simulink model "CC3"  (Simulink 7.5)
settings: Solver=ode45  StartTime=0.0  StopTime=2  RelTol=1e-3
(part 2 of 2)

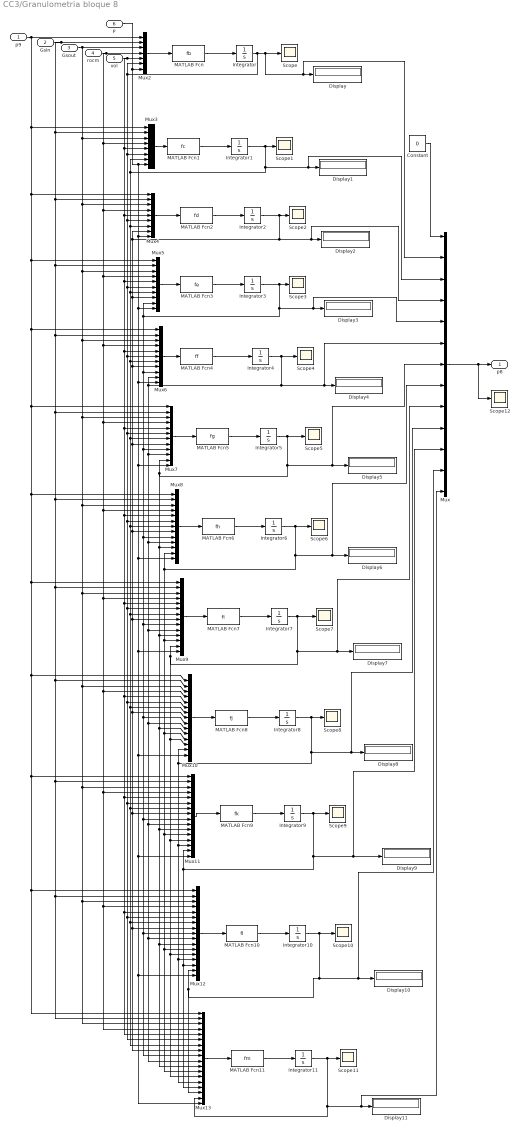
== system CC3/Granulometria bloque 8 ==
  p9 : Inport
  Gsin : Inport  Port=2
  Gsout : Inport  Port=3
  rocm : Inport  Port=4
  vol : Inport  Port=5
  P : Inport  Port=6
  Constant : Constant  Value=0  OutDataType=fixdt(1, 16)  OutScaling=2^0
  Display{,1..11} (12 alike) : Display
  Integrator{,1..11} (12 alike) : Integrator  InitialCondition=0.003
  MATLAB Fcn : MATLABFcn  MATLABFcn=fb
  MATLAB Fcn1 : MATLABFcn  MATLABFcn=fc
  MATLAB Fcn10 : MATLABFcn  MATLABFcn=fl
  MATLAB Fcn11 : MATLABFcn  MATLABFcn=fm
  MATLAB Fcn2 : MATLABFcn  MATLABFcn=fd
  MATLAB Fcn3 : MATLABFcn  MATLABFcn=fe
  MATLAB Fcn4 : MATLABFcn  MATLABFcn=ff
  MATLAB Fcn5 : MATLABFcn  MATLABFcn=fg
  MATLAB Fcn6 : MATLABFcn  MATLABFcn=fh
  MATLAB Fcn7 : MATLABFcn  MATLABFcn=fi
  MATLAB Fcn8 : MATLABFcn  MATLABFcn=fj
  MATLAB Fcn9 : MATLABFcn  MATLABFcn=fk
  Mux : Mux  Inputs=13
  Mux10 : Mux  Inputs=15
  Mux11 : Mux  Inputs=16
  Mux12 : Mux  Inputs=17
  Mux13 : Mux  Inputs=18
  Mux2 : Mux  Inputs=7
  Mux3 : Mux  Inputs=8
  Mux4 : Mux  Inputs=9
  Mux5 : Mux  Inputs=10
  Mux6 : Mux  Inputs=11
  Mux7 : Mux  Inputs=12
  Mux8 : Mux  Inputs=13
  Mux9 : Mux  Inputs=14
  Scope{,1..12} (13 alike) : Scope
      Scope settings: SaveName=ScopeData2
      Scope1 settings: SaveName=ScopeData20
      Scope10 settings: SaveName=ScopeData29
      Scope11 settings: SaveName=ScopeData30
      Scope12 settings: SaveName=ScopeData32
      Scope2 settings: SaveName=ScopeData21
      Scope3 settings: SaveName=ScopeData22
      Scope4 settings: SaveName=ScopeData23
      Scope5 settings: SaveName=ScopeData24
      Scope6 settings: SaveName=ScopeData25
      Scope7 settings: SaveName=ScopeData26
      Scope8 settings: SaveName=ScopeData27
      Scope9 settings: SaveName=ScopeData28
  p8 : Outport  OutDataType=fixdt(1, 16)  OutScaling=2^0
  wires:
  Mux2/1 -> MATLAB Fcn/1
  MATLAB Fcn/1 -> Integrator/1
  Integrator/1 -> Mux2/6, Mux3/6, Mux4/6, Mux5/6, Mux6/6, Mux7/6, Mux8/6, Mux9/6, Mux10/6, Mux11/6, Mux12/6, Mux13/6, Scope/1, Display/1, Mux/2
  p9/1 -> Mux2/1, Mux3/1, Mux4/1, Mux5/1, Mux6/1, Mux7/1, Mux8/1, Mux9/1, Mux10/1, Mux11/1, Mux12/1, Mux13/1
  Gsin/1 -> Mux2/2, Mux3/2, Mux4/2, Mux5/2, Mux6/2, Mux7/2, Mux8/2, Mux9/2, Mux10/2, Mux11/2, Mux12/2, Mux13/2
  Gsout/1 -> Mux2/3, Mux3/3, Mux4/3, Mux5/3, Mux6/3, Mux7/3, Mux8/3, Mux9/3, Mux10/3, Mux11/3, Mux12/3, Mux13/3
  rocm/1 -> Mux2/4, Mux3/4, Mux4/4, Mux5/4, Mux6/4, Mux7/4, Mux8/4, Mux9/4, Mux10/4, Mux11/4, Mux12/4, Mux13/4
  vol/1 -> Mux2/5, Mux3/5, Mux4/5, Mux5/5, Mux6/5, Mux7/5, Mux8/5, Mux9/5, Mux10/5, Mux11/5, Mux12/5, Mux13/5
  Mux3/1 -> MATLAB Fcn1/1
  MATLAB Fcn1/1 -> Integrator1/1
  Integrator1/1 -> Scope1/1, Mux3/7, Mux4/7, Mux5/7, Mux6/7, Mux7/7, Mux8/7, Mux9/7, Mux10/7, Mux11/7, Mux12/7, Mux13/7, Display1/1, Mux/3
  Mux4/1 -> MATLAB Fcn2/1
  MATLAB Fcn2/1 -> Integrator2/1
  Integrator2/1 -> Scope2/1, Mux4/8, Mux5/8, Mux6/8, Mux7/8, Mux8/8, Mux9/8, Mux10/8, Mux11/8, Mux12/8, Mux13/8, Display2/1, Mux/4
  MATLAB Fcn3/1 -> Integrator3/1
  Integrator3/1 -> Scope3/1, Mux5/9, Mux6/9, Mux7/9, Mux8/9, Mux9/9, Mux10/9, Mux11/9, Mux12/9, Mux13/9, Display3/1, Mux/5
  Mux5/1 -> MATLAB Fcn3/1
  Mux6/1 -> MATLAB Fcn4/1
  MATLAB Fcn4/1 -> Integrator4/1
  Integrator4/1 -> Scope4/1, Mux6/10, Mux7/10, Mux8/10, Mux9/10, Mux10/10, Mux11/10, Mux12/10, Mux13/10, Display4/1, Mux/6
  Mux7/1 -> MATLAB Fcn5/1
  MATLAB Fcn5/1 -> Integrator5/1
  Integrator5/1 -> Scope5/1, Mux7/11, Mux8/11, Mux9/11, Mux10/11, Mux11/11, Mux12/11, Mux13/11, Display5/1, Mux/7
  Mux8/1 -> MATLAB Fcn6/1
  MATLAB Fcn6/1 -> Integrator6/1
  Integrator6/1 -> Scope6/1, Mux8/12, Mux9/12, Mux10/12, Mux11/12, Mux12/12, Mux13/12, Display6/1, Mux/8
  Mux9/1 -> MATLAB Fcn7/1
  MATLAB Fcn7/1 -> Integrator7/1
  Integrator7/1 -> Scope7/1, Mux9/13, Mux10/13, Mux11/13, Mux12/13, Mux13/13, Display7/1, Mux/9
  Mux10/1 -> MATLAB Fcn8/1
  MATLAB Fcn8/1 -> Integrator8/1
  Integrator8/1 -> Scope8/1, Mux10/14, Mux11/14, Mux12/14, Mux13/14, Display8/1, Mux/10
  Mux11/1 -> MATLAB Fcn9/1
  MATLAB Fcn9/1 -> Integrator9/1
  Integrator9/1 -> Scope9/1, Mux11/15, Mux12/15, Mux13/15, Display9/1, Mux/11
  Mux12/1 -> MATLAB Fcn10/1
  MATLAB Fcn10/1 -> Integrator10/1
  Integrator10/1 -> Scope10/1, Mux12/16, Mux13/16, Display10/1, Mux/12
  Mux13/1 -> MATLAB Fcn11/1
  MATLAB Fcn11/1 -> Integrator11/1
  Integrator11/1 -> Scope11/1, Mux13/17, Display11/1, Mux/13
  Constant/1 -> Mux/1
  Mux/1 -> p8/1, Scope12/1
  P/1 -> Mux2/7, Mux3/8, Mux4/9, Mux5/10, Mux6/11, Mux7/12, Mux8/13, Mux9/14, Mux10/15, Mux11/16, Mux12/17, Mux13/18

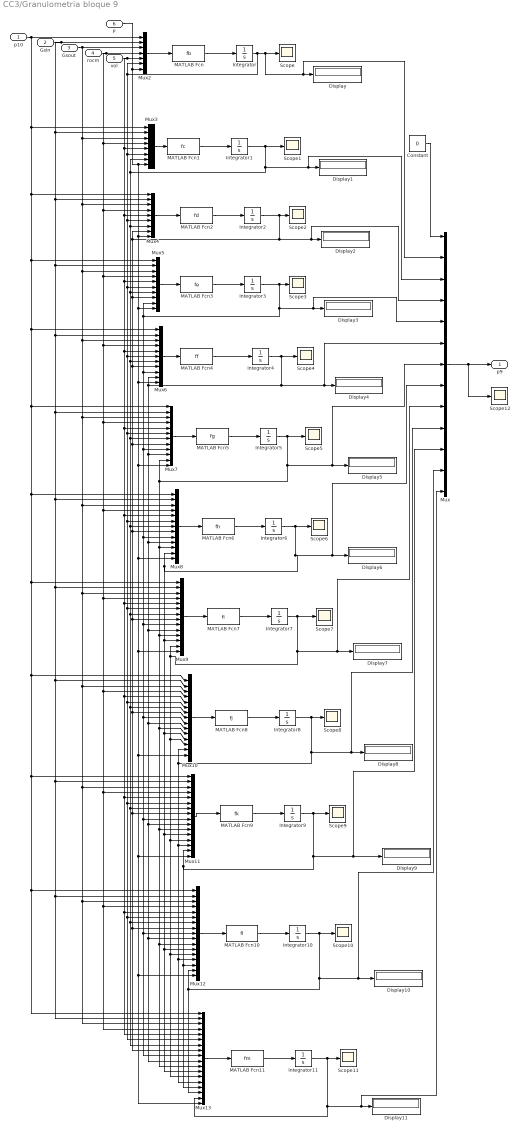
== system CC3/Granulometria bloque 9 ==
  p10 : Inport
  Gsin : Inport  Port=2
  Gsout : Inport  Port=3
  rocm : Inport  Port=4
  vol : Inport  Port=5
  P : Inport  Port=6
  Constant : Constant  Value=0  OutDataType=fixdt(1, 16)  OutScaling=2^0
  Display{,1..11} (12 alike) : Display
  Integrator{,1..11} (12 alike) : Integrator  InitialCondition=0.003
  MATLAB Fcn : MATLABFcn  MATLABFcn=fb
  MATLAB Fcn1 : MATLABFcn  MATLABFcn=fc
  MATLAB Fcn10 : MATLABFcn  MATLABFcn=fl
  MATLAB Fcn11 : MATLABFcn  MATLABFcn=fm
  MATLAB Fcn2 : MATLABFcn  MATLABFcn=fd
  MATLAB Fcn3 : MATLABFcn  MATLABFcn=fe
  MATLAB Fcn4 : MATLABFcn  MATLABFcn=ff
  MATLAB Fcn5 : MATLABFcn  MATLABFcn=fg
  MATLAB Fcn6 : MATLABFcn  MATLABFcn=fh
  MATLAB Fcn7 : MATLABFcn  MATLABFcn=fi
  MATLAB Fcn8 : MATLABFcn  MATLABFcn=fj
  MATLAB Fcn9 : MATLABFcn  MATLABFcn=fk
  Mux : Mux  Inputs=13
  Mux10 : Mux  Inputs=15
  Mux11 : Mux  Inputs=16
  Mux12 : Mux  Inputs=17
  Mux13 : Mux  Inputs=18
  Mux2 : Mux  Inputs=7
  Mux3 : Mux  Inputs=8
  Mux4 : Mux  Inputs=9
  Mux5 : Mux  Inputs=10
  Mux6 : Mux  Inputs=11
  Mux7 : Mux  Inputs=12
  Mux8 : Mux  Inputs=13
  Mux9 : Mux  Inputs=14
  Scope{,1..12} (13 alike) : Scope
      Scope settings: SaveName=ScopeData2
      Scope1 settings: SaveName=ScopeData20
      Scope10 settings: SaveName=ScopeData29
      Scope11 settings: SaveName=ScopeData30
      Scope12 settings: SaveName=ScopeData31
      Scope2 settings: SaveName=ScopeData21
      Scope3 settings: SaveName=ScopeData22
      Scope4 settings: SaveName=ScopeData23
      Scope5 settings: SaveName=ScopeData24
      Scope6 settings: SaveName=ScopeData25
      Scope7 settings: SaveName=ScopeData26
      Scope8 settings: SaveName=ScopeData27
      Scope9 settings: SaveName=ScopeData28
  p9 : Outport  OutDataType=fixdt(1, 16)  OutScaling=2^0
  wires:
  Mux2/1 -> MATLAB Fcn/1
  MATLAB Fcn/1 -> Integrator/1
  Integrator/1 -> Mux2/6, Mux3/6, Mux4/6, Mux5/6, Mux6/6, Mux7/6, Mux8/6, Mux9/6, Mux10/6, Mux11/6, Mux12/6, Mux13/6, Scope/1, Display/1, Mux/2
  p10/1 -> Mux2/1, Mux3/1, Mux4/1, Mux5/1, Mux6/1, Mux7/1, Mux8/1, Mux9/1, Mux10/1, Mux11/1, Mux12/1, Mux13/1
  Gsin/1 -> Mux2/2, Mux3/2, Mux4/2, Mux5/2, Mux6/2, Mux7/2, Mux8/2, Mux9/2, Mux10/2, Mux11/2, Mux12/2, Mux13/2
  Gsout/1 -> Mux2/3, Mux3/3, Mux4/3, Mux5/3, Mux6/3, Mux7/3, Mux8/3, Mux9/3, Mux10/3, Mux11/3, Mux12/3, Mux13/3
  rocm/1 -> Mux2/4, Mux3/4, Mux4/4, Mux5/4, Mux6/4, Mux7/4, Mux8/4, Mux9/4, Mux10/4, Mux11/4, Mux12/4, Mux13/4
  vol/1 -> Mux2/5, Mux3/5, Mux4/5, Mux5/5, Mux6/5, Mux7/5, Mux8/5, Mux9/5, Mux10/5, Mux11/5, Mux12/5, Mux13/5
  Mux3/1 -> MATLAB Fcn1/1
  MATLAB Fcn1/1 -> Integrator1/1
  Mux4/1 -> MATLAB Fcn2/1
  MATLAB Fcn2/1 -> Integrator2/1
  Integrator2/1 -> Scope2/1, Mux4/8, Mux5/8, Mux6/8, Mux7/8, Mux8/8, Mux9/8, Mux10/8, Mux11/8, Mux12/8, Mux13/8, Display2/1, Mux/4
  MATLAB Fcn3/1 -> Integrator3/1
  Integrator3/1 -> Scope3/1, Mux5/9, Mux6/9, Mux7/9, Mux8/9, Mux9/9, Mux10/9, Mux11/9, Mux12/9, Mux13/9, Display3/1, Mux/5
  Mux5/1 -> MATLAB Fcn3/1
  Mux6/1 -> MATLAB Fcn4/1
  MATLAB Fcn4/1 -> Integrator4/1
  Integrator4/1 -> Scope4/1, Mux6/10, Mux7/10, Mux8/10, Mux9/10, Mux10/10, Mux11/10, Mux12/10, Mux13/10, Display4/1, Mux/6
  Mux7/1 -> MATLAB Fcn5/1
  MATLAB Fcn5/1 -> Integrator5/1
  Integrator5/1 -> Scope5/1, Mux7/11, Mux8/11, Mux9/11, Mux10/11, Mux11/11, Mux12/11, Mux13/11, Display5/1, Mux/7
  Mux8/1 -> MATLAB Fcn6/1
  MATLAB Fcn6/1 -> Integrator6/1
  Integrator6/1 -> Scope6/1, Mux8/12, Mux9/12, Mux10/12, Mux11/12, Mux12/12, Mux13/12, Display6/1, Mux/8
  Mux9/1 -> MATLAB Fcn7/1
  MATLAB Fcn7/1 -> Integrator7/1
  Integrator7/1 -> Scope7/1, Mux9/13, Mux10/13, Mux11/13, Mux12/13, Mux13/13, Display7/1, Mux/9
  Mux10/1 -> MATLAB Fcn8/1
  MATLAB Fcn8/1 -> Integrator8/1
  Integrator8/1 -> Scope8/1, Mux10/14, Mux11/14, Mux12/14, Mux13/14, Display8/1, Mux/10
  Mux11/1 -> MATLAB Fcn9/1
  MATLAB Fcn9/1 -> Integrator9/1
  Integrator9/1 -> Scope9/1, Mux11/15, Mux12/15, Mux13/15, Display9/1, Mux/11
  Mux12/1 -> MATLAB Fcn10/1
  MATLAB Fcn10/1 -> Integrator10/1
  Integrator10/1 -> Scope10/1, Mux12/16, Mux13/16, Display10/1, Mux/12
  Mux13/1 -> MATLAB Fcn11/1
  MATLAB Fcn11/1 -> Integrator11/1
  Integrator11/1 -> Scope11/1, Mux13/17, Display11/1, Mux/13
  Constant/1 -> Mux/1
  Mux/1 -> p9/1, Scope12/1
  P/1 -> Mux2/7, Mux3/8, Mux4/9, Mux5/10, Mux6/11, Mux7/12, Mux8/13, Mux9/14, Mux10/15, Mux11/16, Mux12/17, Mux13/18
  Integrator1/1 -> Scope1/1, Mux3/7, Mux4/7, Mux5/7, Mux6/7, Mux7/7, Mux8/7, Mux9/7, Mux10/7, Mux11/7, Mux12/7, Mux13/7, Display1/1, Mux/3

== system CC3/Volumen ==
  Z : Inport
  s0 : Inport  Port=2
  Demux10 : Demux  Outputs=10
  MATLAB Fcn : MATLABFcn  MATLABFcn=Voluumen
  Mux : Mux  Inputs=2
  Vol10 : Outport
  Vol9 : Outport  Port=2
  Vol8 : Outport  Port=3
  Vol7 : Outport  Port=4
  Vol6 : Outport  Port=5
  Vol5 : Outport  Port=6
  Vol4 : Outport  Port=7
  Vol3 : Outport  Port=8
  Vol2 : Outport  Port=9
  Vol1 : Outport  Port=10
  wires:
  Mux/1 -> MATLAB Fcn/1
  MATLAB Fcn/1 -> Demux10/1
  Z/1 -> Mux/1
  s0/1 -> Mux/2
  Demux10/1 -> Vol10/1
  Demux10/2 -> Vol9/1
  Demux10/3 -> Vol8/1
  Demux10/4 -> Vol7/1
  Demux10/5 -> Vol6/1
  Demux10/6 -> Vol5/1
  Demux10/7 -> Vol4/1
  Demux10/8 -> Vol3/1
  Demux10/9 -> Vol2/1
  Demux10/10 -> Vol1/1
